simulink model "FD_YAW_COUPLED"  (R2019b)
settings: Solver=VariableStepAuto  StartTime=0.0  StopTime=10.0  RelTol=1e-3
undefined symbols (not defined in the file): Dt, Jy, k_py, k_yaw
settings Model: Creator=lbend  LastModifiedBy=lbend

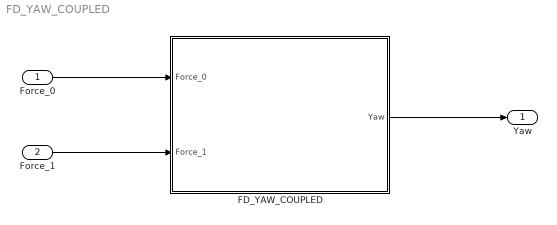
== system FD_YAW_COUPLED ==
  Force_0 : Inport
  "Force_1 " : Inport  Port=2
  FD_YAW_COUPLED : Subsystem
  Yaw : Outport
  wires:
  Force_0/1 -> FD_YAW_COUPLED/1(Force_0)
  "Force_1 "/1 -> FD_YAW_COUPLED/2(Force_1)
  FD_YAW_COUPLED/1(Yaw) -> Yaw/1

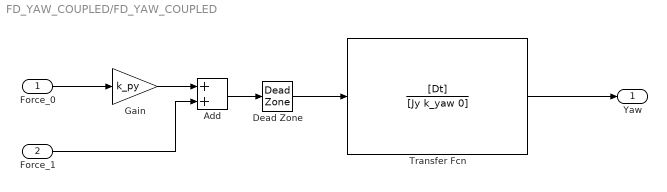
== system FD_YAW_COUPLED/FD_YAW_COUPLED ==
  Force_0 : Inport
  Force_1 : Inport  Port=2
  Add : Sum
  Dead Zone : DeadZone  LowerValue=F_limit_yaw  UpperValue=F_limit_yaw  SaturateOnIntegerOverflow=on
  Gain : Gain  Gain=k_py
  Transfer Fcn : TransferFcn  Numerator=[Dt]  Denominator=[Jy k_yaw 0]
  Yaw : Outport
  wires:
  Transfer Fcn/1 -> Yaw/1
  Dead Zone/1 -> Transfer Fcn/1
  Force_0/1 -> Gain/1
  Add/1 -> Dead Zone/1
  Gain/1 -> Add/1
  Force_1/1 -> Add/2
